simulink model "new_model_Qaurter_Car"  (R2025a)
settings: Solver=FixedStepAuto  StartTime=0.0  StopTime=10.0  FixedStep=0.01  MaxStep=0.01  RelTol=1e-3  AbsTol=1e-6
values from neighbouring files (symbols this model uses):
  ct = 300    [PredictiveSuspensionEnv.m]    (also in simulateTrainedAgent.m; value_constants.m)
  kt = 200000    [PredictiveSuspensionEnv.m]    (also in simulateTrainedAgent.m; value_constants.m)
  msm_sms = 300    [PredictiveSuspensionEnv.m]    (also in simulateTrainedAgent.m; value_constants.m)
  mum_umu = 47    [PredictiveSuspensionEnv.m]    (also in simulateTrainedAgent.m; value_constants.m)
undefined symbols (not defined in the file or in its folder): Cvar, Kvar
libraries: simulink x1
settings Model: LastModifiedBy=Z0187854

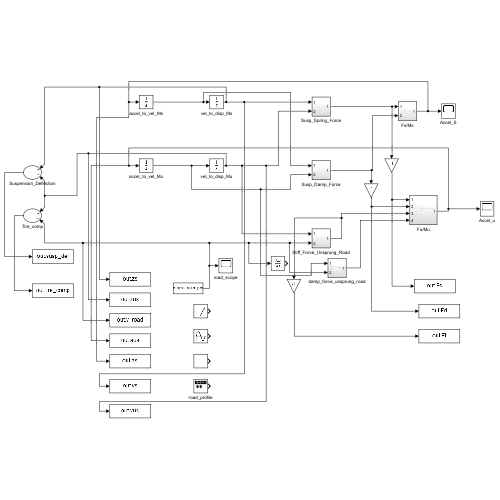
[thumbnail: Simulink's stored preview of the top-level diagram]
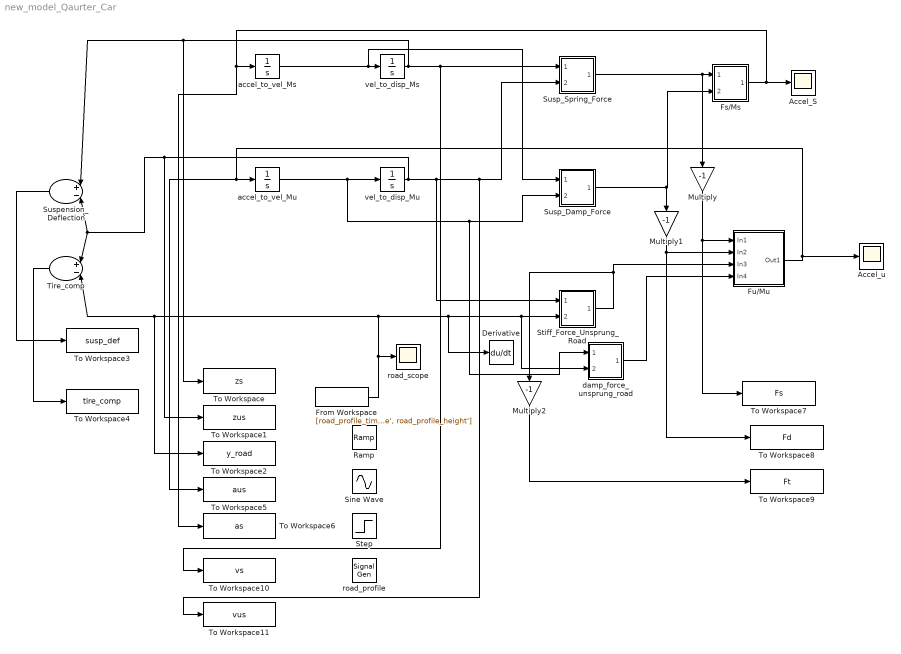
== system new_model_Qaurter_Car ==
  Accel_S : Scope
      settings: ActiveDisplayYMinimum=-1.37296  ActiveDisplayYMaximum=2.14338  DataLoggingVariableName=ScopeData2
  Accel_u : Scope
      settings: ActiveDisplayYMinimum=-9.08155  ActiveDisplayYMaximum=13.48174
  Derivative : Derivative
  From Workspace : FromWorkspace  VariableName=[road_profile_time', road_profile_height']
  Fs/Ms : Subsystem
  Fu/Mu : Subsystem
  Multiply : Gain  Gain=-1
  Multiply1 : Gain  Gain=-1
  Multiply2 : Gain  Gain=-1
  Ramp : simulink/Sources/Ramp  slope=0.5  start=1  InitialOutput=0
  Sine Wave : Sin  SampleTime=0
  Step : Step  After=0.05  SampleTime=0
  Stiff_Force_Unsprung_Road : Subsystem
  Susp_Damp_Force : Subsystem
  Susp_Spring_Force : Subsystem
  Suspension_Deflection : Sum  Inputs=|+-|
  Tire_comp : Sum  Inputs=|+-|
  To Workspace : ToWorkspace  VariableName=zs  SampleTime=-1
  To Workspace1 : ToWorkspace  VariableName=zus  SampleTime=-1
  To Workspace10 : ToWorkspace  VariableName=vs  SampleTime=-1
  To Workspace11 : ToWorkspace  VariableName=vus  SampleTime=-1
  To Workspace2 : ToWorkspace  VariableName=y_road  SampleTime=-1
  To Workspace3 : ToWorkspace  VariableName=susp_def  SaveFormat=Timeseries  SampleTime=-1
  To Workspace4 : ToWorkspace  VariableName=tire_comp  SaveFormat=Timeseries  SampleTime=-1
  To Workspace5 : ToWorkspace  VariableName=aus  SampleTime=-1
  To Workspace6 : ToWorkspace  VariableName=as  SampleTime=-1
  To Workspace7 : ToWorkspace  VariableName=Fs  SampleTime=-1
  To Workspace8 : ToWorkspace  VariableName=Fd  SampleTime=-1
  To Workspace9 : ToWorkspace  VariableName=Ft  SampleTime=-1
  accel_to_vel_Ms : Integrator
  accel_to_vel_Mu : Integrator
  damp_force_unsprung_road : Subsystem
  road_profile : SignalGenerator  Amplitude=0.2  Frequency=0.2
  road_scope : Scope
      settings: ActiveDisplayYMinimum=-0.25  ActiveDisplayYMaximum=0.25
  vel_to_disp_Ms : Integrator
  vel_to_disp_Mu : Integrator
  wires:
  accel_to_vel_Ms/1 -> Susp_Damp_Force/1(In1), vel_to_disp_Ms/1
  accel_to_vel_Mu/1 -> Susp_Damp_Force/2(In2), damp_force_unsprung_road/1(In1), vel_to_disp_Mu/1
  vel_to_disp_Ms/1 -> Suspension_Deflection/1, To Workspace/1, To Workspace10/1, Susp_Spring_Force/1(In1)
  vel_to_disp_Mu/1 -> Suspension_Deflection/2, Tire_comp/1, To Workspace1/1, Stiff_Force_Unsprung_Road/1(In1), To Workspace11/1, Susp_Spring_Force/2(In2)
  Susp_Spring_Force/1(Out1) -> Multiply/1, Fs/Ms/1(In1)
  Susp_Damp_Force/1(Out1) -> Fs/Ms/2(In2), Multiply1/1
  Fs/Ms/1(Out1) -> Accel_S/1, To Workspace6/1, accel_to_vel_Ms/1
  Stiff_Force_Unsprung_Road/1(Out1) -> Multiply2/1, Fu/Mu/3(In3)
  Fu/Mu/1(Out1) -> Accel_u/1, To Workspace5/1, accel_to_vel_Mu/1
  Multiply/1 -> To Workspace7/1, Fu/Mu/1(In1)
  Multiply1/1 -> To Workspace8/1, Fu/Mu/2(In2)
  Suspension_Deflection/1 -> To Workspace3/1
  Tire_comp/1 -> To Workspace4/1
  Multiply2/1 -> To Workspace9/1
  From Workspace/1 -> To Workspace2/1, Tire_comp/2, Derivative/1, Stiff_Force_Unsprung_Road/2(In2), damp_force_unsprung_road/2(In2), road_scope/1
  damp_force_unsprung_road/1(Out1) -> Fu/Mu/4(In4)

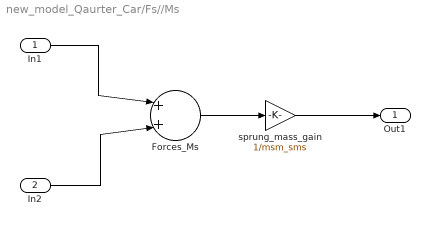
== system new_model_Qaurter_Car/Fs//Ms ==
  In1 : Inport
  In2 : Inport  Port=2
  Forces_Ms : Sum  Inputs=|++|
  sprung_mass_gain : Gain  Gain=1/msm_sms
  Out1 : Outport
  wires:
  Forces_Ms/1 -> sprung_mass_gain/1
  In1/1 -> Forces_Ms/1
  sprung_mass_gain/1 -> Out1/1
  In2/1 -> Forces_Ms/2

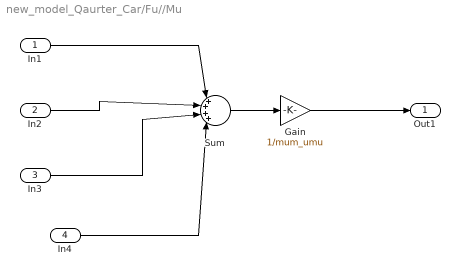
== system new_model_Qaurter_Car/Fu//Mu ==
  In1 : Inport
  In2 : Inport  Port=2
  In3 : Inport  Port=3
  In4 : Inport  Port=4
  Gain : Gain  Gain=1/mum_umu
  Sum : Sum  Inputs=|++++|
  Out1 : Outport
  wires:
  Sum/1 -> Gain/1
  In3/1 -> Sum/3
  Gain/1 -> Out1/1
  In2/1 -> Sum/2
  In1/1 -> Sum/1
  In4/1 -> Sum/4

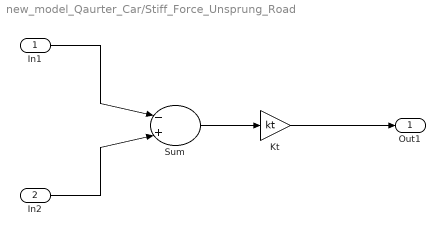
== system new_model_Qaurter_Car/Stiff_Force_Unsprung_Road ==
  In1 : Inport
  In2 : Inport  Port=2
  Kt : Gain  Gain=kt
  Sum : Sum  Inputs=|-+|
  Out1 : Outport
  wires:
  Sum/1 -> Kt/1
  Kt/1 -> Out1/1
  In2/1 -> Sum/2
  In1/1 -> Sum/1

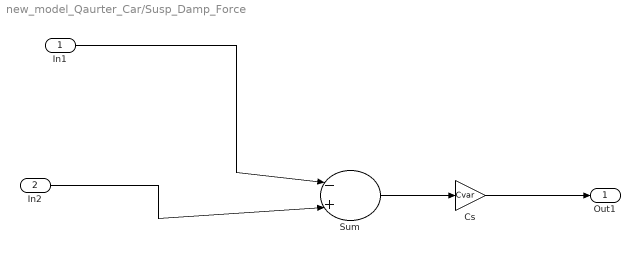
== system new_model_Qaurter_Car/Susp_Damp_Force ==
  In1 : Inport
  In2 : Inport  Port=2
  Cs : Gain  Gain=Cvar
  Sum : Sum  Inputs=|-+|
  Out1 : Outport
  wires:
  Sum/1 -> Cs/1
  In2/1 -> Sum/2
  Cs/1 -> Out1/1
  In1/1 -> Sum/1

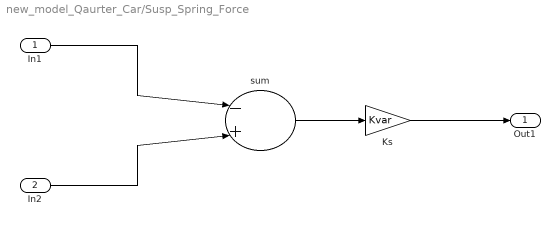
== system new_model_Qaurter_Car/Susp_Spring_Force ==
  In1 : Inport
  In2 : Inport  Port=2
  Ks : Gain  Gain=Kvar
  sum : Sum  Inputs=|-+|
  Out1 : Outport
  wires:
  sum/1 -> Ks/1
  In2/1 -> sum/2
  In1/1 -> sum/1
  Ks/1 -> Out1/1

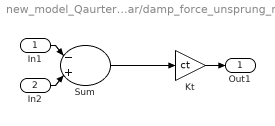
== system new_model_Qaurter_Car/damp_force_unsprung_road ==
  In1 : Inport
  In2 : Inport  Port=2
  Kt : Gain  Gain=ct
  Sum : Sum  Inputs=|-+|
  Out1 : Outport
  wires:
  Sum/1 -> Kt/1
  In1/1 -> Sum/1
  In2/1 -> Sum/2
  Kt/1 -> Out1/1
